simulink model "my_simulation"  (R2024b)
settings: Solver=VariableStepAuto  StartTime=0.0  StopTime=10.0  RelTol=1e-3
settings Model: Creator=xinxing  LastModifiedBy=xinxing

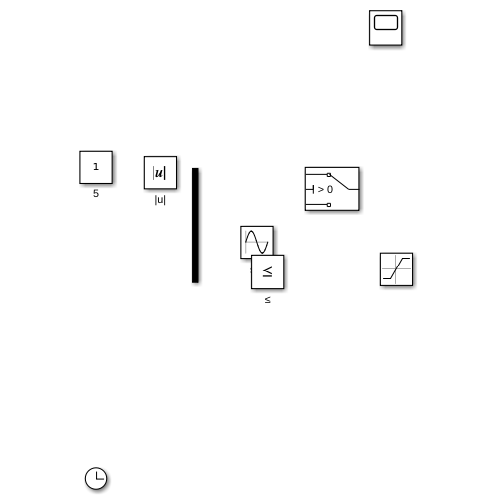
[thumbnail: Simulink's stored preview of the top-level diagram]
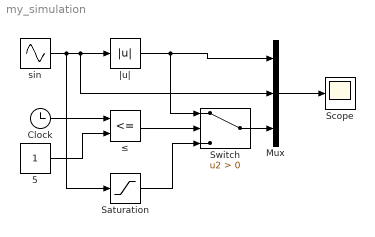
== system my_simulation ==
  5 : Constant
  Clock : Clock
  Mux : Mux  Inputs=3
  Saturation : Saturate
  Scope : Scope
  Switch : Switch  Criteria=u2 > Threshold  SaturateOnIntegerOverflow=off  InputSameDT=off
  sin : Sin  SampleTime=0
  |u| : Abs  SaturateOnIntegerOverflow=off
  ≤ : RelationalOperator  Operator=<=  OutDataTypeStr=boolean  RndMeth=Simplest  InputSameDT=off
  wires:
  Switch/1 -> Mux/3
  Mux/1 -> Scope/1
  Saturation/1 -> Switch/3
  ≤/1 -> Switch/2
  |u|/1 -> Switch/1, Mux/1
  5/1 -> ≤/2
  Clock/1 -> ≤/1
  sin/1 -> |u|/1, Mux/2, Saturation/1
